simulink model "SOH_relaxed_voltage_estimator"  (R2024a)
settings: Solver=FixedStepAuto  StartTime=0.0  StopTime=3600  FixedStep=1  RelTol=1e-3
values from neighbouring files (symbols this model uses):
  BATTERY_MODULE_CAPACITY_AH = 51.0    [ParametersDataDictionary.sldd]    (also in SOXDictionary.sldd; SOXDictionaryGotion.sldd = 116.0
  OCV_SOC : value not decoded    [CellDictionary.sldd]
  OCV_T : value not decoded    [CellDictionary.sldd]
  OCV_V = 3.089975 3.1958025155770748 3.2700856729308603 3.3269062967469782 3.3701558672655878 3.3935018471075473 3.4031249999999997 3.4106750000000003 3.417975 3.4255687342956502 3.4340073517474323 3.44463535689108 3.4571649659479133 3.4695529273207848 3.481325 3.49315 3.5048949462107366 3.5157966467267432 3.5254768755401917 3.534725 3.543897510782176 3.5528756373568848 3.5611426187731481 3.5686 3.575725 3    [CellDictionary.sldd]    (also in Gotion116CellDictionary.sldd; ParametersDataDictionary.sldd = 3.426 3.511 3.595 3.627 3.656 3.705 3.785 3.893 3.955 4.054 ; SOXDictionary.sldd = 3.426 3.511 3.595 3.627 3.656 3.705 3.785 3.893 3.955 4.054 ; SOXDictionaryGotion.sldd = 2.8 3.089975 3.1958025155770748 3.2700856729308603 3.3269062)
  SOH_DOD_THRESHOLD = 0.1    [SOXDictionaryGotion.sldd]
  SOH_ESTIM_INIT = 1.0    [SOXDictionaryGotion.sldd]
  SOH_LPF_ALPHA = 0.1    [SOXDictionaryGotion.sldd]
  SOH_REST_CURRENT_THRESHOLD = 0.05    [SOXDictionaryGotion.sldd]
  SOH_REST_TIME_THRESHOLD = 3600.0    [SOXDictionaryGotion.sldd]
  SOH_TIMESTEP = 1.0    [SOXDictionaryGotion.sldd]
undefined symbols (not defined in the file or in its folder): DiscIntNeverNeededParam
libraries: simulink x2
settings Model: DataDictionary=SOXDictionaryGotion.sldd  SimulationMode=accelerator  Creator=mmackenzie  LastModifiedBy=mmackenzie
settings DebuggingCC: ParamPrecisionLossAbsoluteDiffThreshold=1e-8  ParamPrecisionLossRelativeDiffThreshold=1e-6

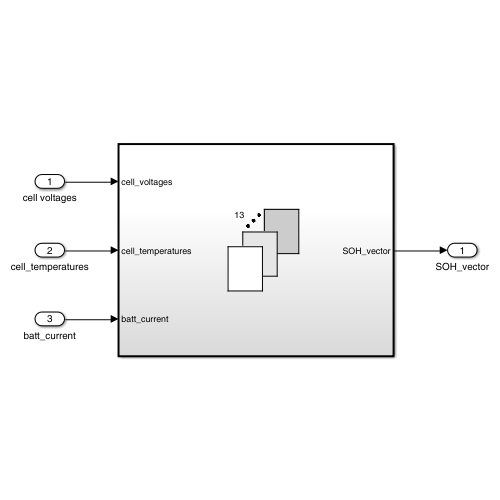
[thumbnail: Simulink's stored preview of the top-level diagram]
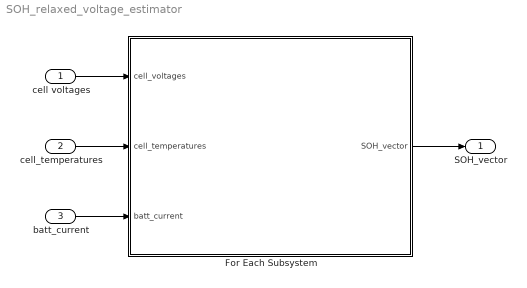
== system SOH_relaxed_voltage_estimator ==
  cell voltages : Inport  OutDataTypeStr=single  PortDimensions=N_CELL_VOLTAGE
  cell_temperatures : Inport  Port=2  OutDataTypeStr=single  PortDimensions=N_CELL_VOLTAGE
  batt_current : Inport  Port=3  OutDataTypeStr=single
  For Each Subsystem : Subsystem  TreatAsAtomicUnit=on
  SOH_vector : Outport
  wires:
  For Each Subsystem/1(SOH_vector) -> SOH_vector/1
  cell voltages/1 -> For Each Subsystem/1(cell_voltages)
  batt_current/1 -> For Each Subsystem/3(batt_current)
  cell_temperatures/1 -> For Each Subsystem/2(cell_temperatures)

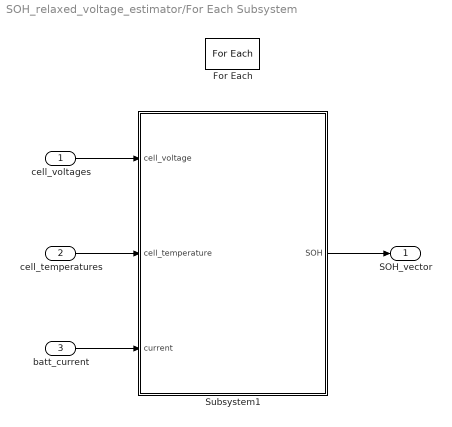
== system SOH_relaxed_voltage_estimator/For Each Subsystem ==
  cell_voltages : Inport  Partition=on  PartitionDimension=1  PartitionWidth=1  PartitionOffset=0
  cell_temperatures : Inport  Port=2  Partition=on  PartitionDimension=1  PartitionWidth=1  PartitionOffset=0
  batt_current : Inport  Port=3
  For Each : ForEach  DisableCoverage=on
  Subsystem1 : Subsystem
  SOH_vector : Outport  ConcatenationDimension=1
  wires:
  Subsystem1/1(SOH) -> SOH_vector/1
  batt_current/1 -> Subsystem1/3(current)
  cell_temperatures/1 -> Subsystem1/2(cell_temperature)
  cell_voltages/1 -> Subsystem1/1(cell_voltage)

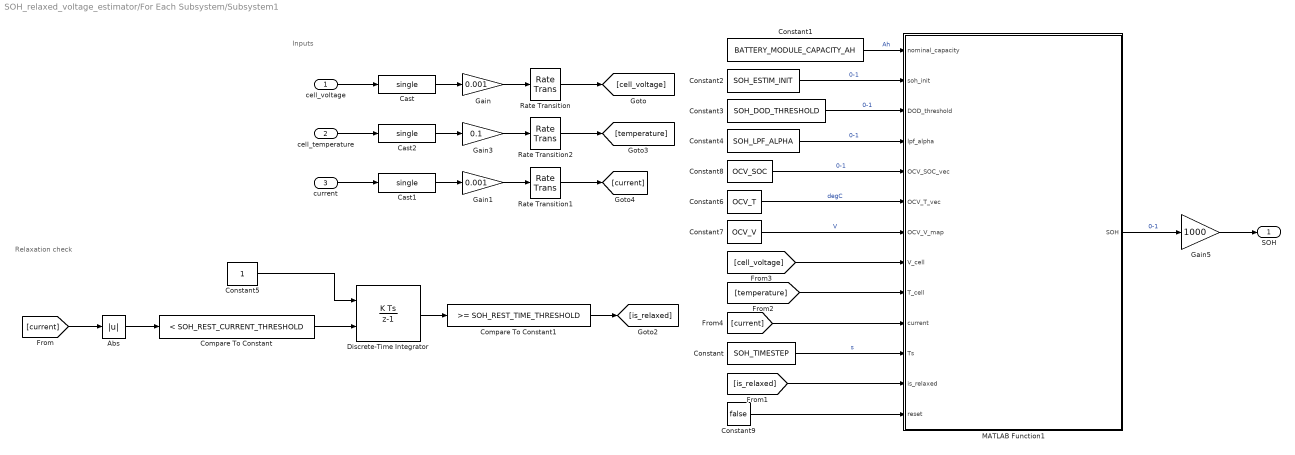
== system SOH_relaxed_voltage_estimator/For Each Subsystem/Subsystem1 ==
  note: Relaxation check
  note: Inputs
  cell_voltage : Inport
  cell_temperature : Inport  Port=2
  current : Inport  Port=3
  Abs : Abs  SaturateOnIntegerOverflow=off
  Cast : DataTypeConversion  OutDataTypeStr=single  SaturateOnIntegerOverflow=off  RndMeth=Floor
  Cast1 : DataTypeConversion  OutDataTypeStr=single  SaturateOnIntegerOverflow=off  RndMeth=Floor
  Cast2 : DataTypeConversion  OutDataTypeStr=single  SaturateOnIntegerOverflow=off  RndMeth=Floor
  Compare To Constant : simulink/Logic and Bit Operations/Compare To Constant  relop=<  const=SOH_REST_CURRENT_THRESHOLD  OutDataTypeStr=boolean
  Compare To Constant1 : simulink/Logic and Bit Operations/Compare To Constant  relop=>=  const=SOH_REST_TIME_THRESHOLD  OutDataTypeStr=boolean
  Constant : Constant  Value=SOH_TIMESTEP
  Constant1 : Constant  Value=BATTERY_MODULE_CAPACITY_AH
  Constant2 : Constant  Value=SOH_ESTIM_INIT
  Constant3 : Constant  Value=SOH_DOD_THRESHOLD
  Constant4 : Constant  Value=SOH_LPF_ALPHA
  Constant5 : Constant
  Constant6 : Constant  Value=OCV_T
  Constant7 : Constant  Value=OCV_V
  Constant8 : Constant  Value=OCV_SOC
  Constant9 : Constant  Value=false
  Discrete-Time Integrator : DiscreteIntegrator  ExternalReset=falling  SampleTime=-1  ICPrevOutput=DiscIntNeverNeededParam  ICPrevScaledInput=DiscIntNeverNeededParam
  Gain : Gain  Gain=0.001
  Gain1 : Gain  Gain=0.001
  Gain3 : Gain  Gain=0.1
  Gain5 : Gain  Gain=1000
  MATLAB Function1 : MATLAB Function  TreatAsAtomicUnit=on
  Rate Transition : RateTransition  Integrity=off  OutPortSampleTime=1
  Rate Transition1 : RateTransition  Integrity=off  OutPortSampleTime=1
  Rate Transition2 : RateTransition  Integrity=off  OutPortSampleTime=1
  SOH : Outport
  wires:
  Rate Transition1/1 -> [current]
  Gain5/1 -> SOH/1
  Gain1/1 -> Rate Transition1/1
  current/1 -> Cast1/1
  Cast1/1 -> Gain1/1
  Constant/1 -> MATLAB Function1/11(Ts)  "s"
  MATLAB Function1/1(SOH) -> Gain5/1  "0-1"
  Constant2/1 -> MATLAB Function1/2(soh_init)  "0-1"
  [is_relaxed] -> MATLAB Function1/12(is_relaxed)
  Constant1/1 -> MATLAB Function1/1(nominal_capacity)  "Ah"
  Constant3/1 -> MATLAB Function1/3(DOD_threshold)  "0-1"
  Constant4/1 -> MATLAB Function1/4(lpf_alpha)  "0-1"
  Constant8/1 -> MATLAB Function1/5(OCV_SOC_vec)  "0-1"
  Constant6/1 -> MATLAB Function1/6(OCV_T_vec)  "degC"
  Constant7/1 -> MATLAB Function1/7(OCV_V_map)  "V"
  cell_voltage/1 -> Cast/1
  Rate Transition/1 -> [cell_voltage]
  Cast/1 -> Gain/1
  Gain/1 -> Rate Transition/1
  cell_temperature/1 -> Cast2/1
  Rate Transition2/1 -> [temperature]
  Gain3/1 -> Rate Transition2/1
  Cast2/1 -> Gain3/1
  [temperature] -> MATLAB Function1/9(T_cell)
  [cell_voltage] -> MATLAB Function1/8(V_cell)
  [current] -> MATLAB Function1/10(current)
  Constant9/1 -> MATLAB Function1/13(reset)
  [current] -> Abs/1
  Abs/1 -> Compare To Constant/1
  Compare To Constant/1 -> Discrete-Time Integrator/2
  Discrete-Time Integrator/1 -> Compare To Constant1/1
  Compare To Constant1/1 -> [is_relaxed]
  Constant5/1 -> Discrete-Time Integrator/1

== matlab function SOH_relaxed_voltage_estimator/For Each Subsystem/Subsystem1/MATLAB Function1 ==
  data: nominal_capacity input; soh_init input; DOD_threshold input; lpf_alpha input; OCV_SOC_vec input; OCV_T_vec input; OCV_V_map input; V_cell input; T_cell input; current input; Ts input; is_relaxed input; SOH output; reset input
function SOH  = SOH_Snapshot_Estimator(nominal_capacity, soh_init, DOD_threshold, lpf_alpha, OCV_SOC_vec, OCV_T_vec, OCV_V_map, V_cell, T_cell, current, Ts, is_relaxed, reset)
    % is_relaxed: Boolean from the BMS logic (e.g., |I| < 0.05A for 60 mins)
    % V_relaxed: The voltage measured during the relaxation state
    
    persistent start_soc accum_Ah has_start_point current_SOH
    
    % Initialisation
    if isempty(current_SOH) || reset
        current_SOH = single(soh_init);
        start_soc = single(0);
        accum_Ah = single(0);
        has_start_point = false;
    end

    % Temperature slicing
    T_clamped = max(OCV_T_vec(1), min(OCV_T_vec(end), T_cell));
    OCV_at_T = interp2(OCV_T_vec, OCV_SOC_vec, OCV_V_map, T_clamped, OCV_SOC_vec, 'linear');

    % Start snapshot
    if is_relaxed && ~has_start_point
        % Inverse OCV lookup: V -> SOC
        start_soc = interp1(OCV_at_T, OCV_SOC_vec, V_cell, 'linear');
        accum_Ah = single(0);
        has_start_point = true;
    end

    % Current integration
    if ~is_relaxed && has_start_point
        accum_Ah = accum_Ah + (current * Ts / 3600);
    end

    % End snapshot
    if is_relaxed && has_start_point
        end_soc = interp1(OCV_at_T, OCV_SOC_vec, V_cell, 'linear');
        delta_soc = abs(end_soc - start_soc);
        
        % Only update if the delta SOC is larger than the DOD threshold
        if delta_soc > DOD_threshold
            measured_cap = abs(accum_Ah) / delta_soc;
            
            % Low-pass filter to update the SOH slowly
            alpha = single(lpf_alpha);
            new_SOH = measured_cap / nominal_capacity;
            
            current_SOH = (1 - alpha) * current_SOH + alpha * new_SOH;
            
            % Reset for the next major cycle
            has_start_point = false;
        end
    end

    SOH = current_SOH;
end
